simulink model "sampleModel1985"  (R2023a)
settings: Solver=VariableStepAuto  StartTime=0.0  StopTime=10.0  RelTol=1e-3
libraries: hdlsllib x2
settings Model: Creator=user1  LastModifiedBy=user1

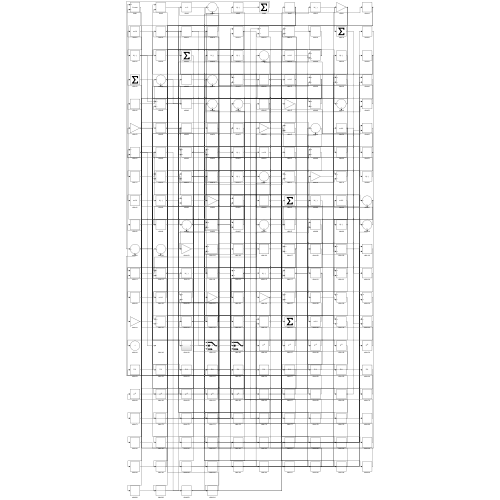
[thumbnail: Simulink's stored preview of the top-level diagram]
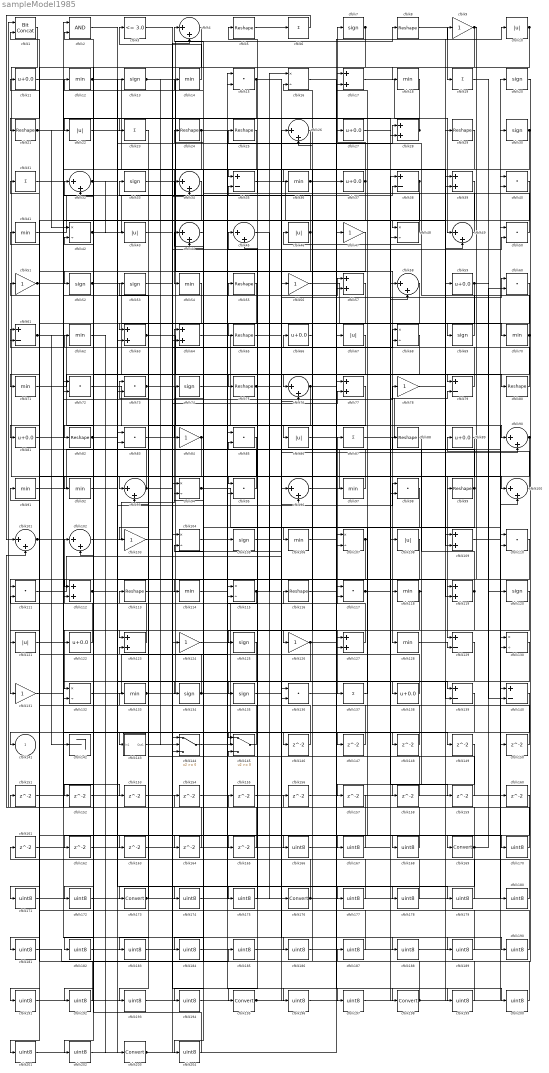
== system sampleModel1985 ==
  cfblk1 : hdlsllib/Logic and Bit Operations/Bit Concat  numInputs=2
  cfblk{10,22,43,46,67,86,108,121} (8 alike) : Abs  SaturateOnIntegerOverflow=off
  cfblk{4,26,32,34,44..45,49,58,76,90,93,96,100..102} (15 alike) : Sum  Inputs=|++
  cfblk{9,47,51,56,78,84,103,124,126,131} (10 alike) : Gain
  cfblk{16,42,48,68,94,104,107,115,130,132} (10 alike) : Product  Inputs=*/  RndMeth=Zero  SaturateOnIntegerOverflow=on
  cfblk{7,13,20,30,33,52..53,69,74,105,120,125,134..135} (14 alike) : Signum
  cfblk{12,14,18,36,41,54,62,70..71,91..92,97,106,114,118,128,133} (17 alike) : MinMax
  cfblk{17,28,39,57,63..64,77,109,112,119,123,127} (12 alike) : Sum
  cfblk{11,27,37,59,66,81,89,122,138} (9 alike) : Bias  Bias=0.0  SaturateOnIntegerOverflow=off
  cfblk{15,40,50,60,72..73,83,85,95,98,110..111,117,136} (14 alike) : DotProduct  OutDataTypeStr=Inherit: Inherit via internal rule
  cfblk{5,8,21,24..25,29,55,65,75,80,82,88,99,113,116} (15 alike) : Reshape
  cfblk{35,38,61,79,129,139..140} (7 alike) : Sum  Inputs=+-
  cfblk{6,19,23,31,87,137} (6 alike) : Sum  Inputs=+
  cfblk142 : Terminator
  cfblk143 : Subsystem
      settings: LibrarySourceBlock=|
      | hdlsllib/Ports &
      | Subsystems/Subsystem
  cfblk144 : Switch  SaturateOnIntegerOverflow=off  InputSameDT=off
  cfblk145 : Switch  SaturateOnIntegerOverflow=off  InputSameDT=off
  cfblk{146..165} (20 alike) : Delay  SampleTime=1
  cfblk{166..168,170..172,174..175,177..194,196..197,199..202,204} (33 alike) : DataTypeConversion  OutDataTypeStr=uint8  SaturateOnIntegerOverflow=off  RndMeth=Floor
  cfblk{169,173,176,195,198,203} (6 alike) : DataTypeConversion  SaturateOnIntegerOverflow=off  RndMeth=Floor
  cfblk2 : Logic  AllPortsSameDT=off  OutDataTypeStr=boolean
  cfblk3 : hdlsllib/Logic and Bit Operations/Compare To Constant  relop=<=  const=3.0  OutDataTypeStr=boolean
  cfblk141 : Outport  VectorParamsAs1DForOutWhenUnconnected=off
  wires:
  cfblk113/1 -> cfblk8/1
  cfblk19/1 -> cfblk120/1
  cfblk83/1 -> cfblk66/1
  cfblk25/1 -> cfblk54/1
  cfblk139/1 -> cfblk141/1
  cfblk5/1 -> cfblk6/1
  cfblk119/1 -> cfblk137/1, cfblk88/1
  cfblk52/1 -> cfblk69/1, cfblk80/1
  cfblk56/1 -> cfblk70/1
  cfblk13/1 -> cfblk128/1, cfblk144/2
  cfblk60/1 -> cfblk79/1
  cfblk61/1 -> cfblk86/1, cfblk143/1(In1), cfblk142/1
  cfblk104/1 -> cfblk198/1
  cfblk99/1 -> cfblk42/2, cfblk147/1
  cfblk122/1 -> cfblk102/1
  cfblk78/1 -> cfblk10/1
  cfblk49/1 -> cfblk12/1
  cfblk1/1 -> cfblk93/1
  cfblk102/1 -> cfblk64/1
  cfblk11/1 -> cfblk35/1
  cfblk117/1 -> cfblk79/2, cfblk149/1
  cfblk46/1 -> cfblk33/1, cfblk75/1, cfblk65/1
  cfblk6/1 -> cfblk101/1
  cfblk118/1 -> cfblk157/1, cfblk158/1
  cfblk77/1 -> cfblk123/1
  cfblk57/1 -> cfblk103/1
  cfblk37/1 -> cfblk7/1, cfblk194/1
  cfblk73/1 -> cfblk178/1, cfblk180/1, cfblk197/1
  cfblk92/1 -> cfblk28/1
  cfblk48/1 -> cfblk4/1
  cfblk127/1 -> cfblk87/1
  cfblk84/1 -> cfblk102/2, cfblk44/2, cfblk191/1
  cfblk120/1 -> cfblk132/1
  cfblk53/1 -> cfblk94/1
  cfblk45/1 -> cfblk176/1
  cfblk137/1 -> cfblk17/1
  cfblk69/1 -> cfblk46/1
  cfblk66/1 -> cfblk106/1
  cfblk63/1 -> cfblk96/1, cfblk35/2
  cfblk111/1 -> cfblk96/2
  cfblk28/1 -> cfblk22/1, cfblk23/1
  cfblk71/1 -> cfblk76/1
  cfblk79/1 -> cfblk44/1
  cfblk76/1 -> cfblk115/2, cfblk9/1
  cfblk144/1 -> cfblk67/1
  cfblk12/1 -> cfblk144/1, cfblk117/2
  cfblk133/1 -> cfblk56/1, cfblk77/2
  cfblk132/1 -> cfblk105/1
  cfblk15/1 -> cfblk82/1, cfblk162/1, cfblk170/1
  cfblk24/1 -> cfblk83/2, cfblk36/1
  cfblk131/1 -> cfblk78/1
  cfblk17/1 -> cfblk49/1
  cfblk88/1 -> cfblk118/1
  cfblk80/1 -> cfblk61/1
  cfblk95/1 -> cfblk32/1
  cfblk134/1 -> cfblk94/2, cfblk73/1, cfblk53/1, cfblk116/1, cfblk32/2
  cfblk70/1 -> cfblk25/1, cfblk95/1
  cfblk31/1 -> cfblk169/1
  cfblk115/1 -> cfblk26/1, cfblk111/2, cfblk16/1
  cfblk96/1 -> cfblk39/1
  cfblk51/1 -> cfblk153/1, cfblk186/1
  cfblk75/1 -> cfblk60/1, cfblk119/2
  cfblk91/1 -> cfblk30/1
  cfblk35/1 -> cfblk49/2
  cfblk124/1 -> cfblk117/1
  cfblk9/1 -> cfblk112/1, cfblk18/1, cfblk119/1
  cfblk103/1 -> cfblk68/1
  cfblk4/1 -> cfblk122/1
  cfblk21/1 -> cfblk48/1, cfblk42/1, cfblk28/2
  cfblk39/1 -> cfblk72/2
  cfblk7/1 -> cfblk64/2, cfblk63/2, cfblk152/1
  cfblk143/1(Out1) -> cfblk68/2
  cfblk72/1 -> cfblk97/1
  cfblk59/1 -> cfblk134/1, cfblk140/2, cfblk63/1
  cfblk90/1 -> cfblk129/1, cfblk111/1
  cfblk33/1 -> cfblk48/2
  cfblk89/1 -> cfblk138/1
  cfblk41/1 -> cfblk4/2
  cfblk58/1 -> cfblk195/1
  cfblk108/1 -> cfblk131/1
  cfblk29/1 -> cfblk84/1
  cfblk26/1 -> cfblk145/1
  cfblk94/1 -> cfblk140/1, cfblk168/1
  cfblk54/1 -> cfblk112/2
  cfblk100/1 -> cfblk89/1
  cfblk101/1 -> cfblk55/1, cfblk34/1
  cfblk82/1 -> cfblk139/1, cfblk172/1
  cfblk85/1 -> cfblk173/1
  cfblk93/1 -> cfblk50/2, cfblk135/1, cfblk41/1
  cfblk34/1 -> cfblk71/1
  cfblk107/1 -> cfblk17/2, cfblk121/1, cfblk174/1
  cfblk121/1 -> cfblk57/1
  cfblk128/1 -> cfblk129/2
  cfblk67/1 -> cfblk92/1
  cfblk22/1 -> cfblk109/1
  cfblk42/1 -> cfblk38/2, cfblk100/1
  cfblk62/1 -> cfblk203/1
  cfblk38/1 -> cfblk125/1, cfblk73/2, cfblk52/1
  cfblk8/1 -> cfblk19/1
  cfblk32/1 -> cfblk43/1, cfblk177/1
  cfblk16/1 -> cfblk107/1
  cfblk3/1 -> cfblk124/1
  cfblk123/1 -> cfblk113/1
  cfblk98/1 -> cfblk114/1
  cfblk145/1 -> cfblk133/1
  cfblk126/1 -> cfblk107/2, cfblk164/1
  cfblk138/1 -> cfblk11/1
  cfblk87/1 -> cfblk59/1
  cfblk129/1 -> cfblk132/2
  cfblk55/1 -> cfblk81/1
  cfblk36/1 -> cfblk109/2, cfblk139/2
  cfblk50/1 -> cfblk5/1
  cfblk14/1 -> cfblk3/1
  cfblk30/1 -> cfblk126/1, cfblk95/2
  cfblk10/1 -> cfblk99/1, cfblk21/1
  cfblk64/1 -> cfblk90/1
  cfblk112/1 -> cfblk98/1, cfblk175/1
  cfblk114/1 -> cfblk127/2
  cfblk97/1 -> cfblk14/1
  cfblk65/1 -> cfblk90/2
  cfblk81/1 -> cfblk146/1
  cfblk146/1 -> cfblk1/2
  cfblk147/1 -> cfblk127/1
  cfblk105/1 -> cfblk148/1
  cfblk148/1 -> cfblk38/1
  cfblk109/1 -> cfblk150/1
  cfblk150/1 -> cfblk26/2
  cfblk151/1 -> cfblk72/1
  cfblk152/1 -> cfblk145/2
  cfblk153/1 -> cfblk76/2
  cfblk154/1 -> cfblk115/1
  cfblk155/1 -> cfblk50/1
  cfblk156/1 -> cfblk98/2
  cfblk157/1 -> cfblk101/2
  cfblk158/1 -> cfblk145/3
  cfblk27/1 -> cfblk159/1
  cfblk159/1 -> cfblk93/2
  cfblk161/1 -> cfblk83/1
  cfblk162/1 -> cfblk34/2
  cfblk68/1 -> cfblk163/1
  cfblk163/1 -> cfblk57/2
  cfblk164/1 -> cfblk61/2
  cfblk140/1 -> cfblk165/1
  cfblk165/1 -> cfblk1/1
  cfblk2/1 -> cfblk166/1
  cfblk166/1 -> cfblk108/1
  cfblk149/1 -> cfblk167/1
  cfblk167/1 -> cfblk2/1
  cfblk168/1 -> cfblk2/2
  cfblk169/1 -> cfblk60/2, cfblk24/1, cfblk183/1
  cfblk170/1 -> cfblk31/1
  cfblk160/1 -> cfblk171/1
  cfblk171/1 -> cfblk15/1
  cfblk172/1 -> cfblk160/1
  cfblk173/1 -> cfblk15/2, cfblk123/2, cfblk27/1
  cfblk174/1 -> cfblk85/1
  cfblk175/1 -> cfblk85/2
  cfblk176/1 -> cfblk156/1, cfblk155/1
  cfblk177/1 -> cfblk45/1
  cfblk178/1 -> cfblk45/2
  cfblk74/1 -> cfblk179/1
  cfblk179/1 -> cfblk51/1
  cfblk180/1 -> cfblk74/1
  cfblk40/1 -> cfblk181/1
  cfblk125/1 -> cfblk182/1
  cfblk182/1 -> cfblk40/1
  cfblk183/1 -> cfblk40/2
  cfblk110/1 -> cfblk184/1
  cfblk184/1 -> cfblk37/1
  cfblk181/1 -> cfblk185/1
  cfblk185/1 -> cfblk110/1
  cfblk186/1 -> cfblk110/2
  cfblk20/1 -> cfblk187/1
  cfblk187/1 -> cfblk161/1
  cfblk106/1 -> cfblk188/1
  cfblk188/1 -> cfblk20/1
  cfblk136/1 -> cfblk189/1
  cfblk189/1 -> cfblk154/1
  cfblk135/1 -> cfblk190/1
  cfblk190/1 -> cfblk136/1
  cfblk191/1 -> cfblk136/2
  cfblk130/1 -> cfblk192/1
  cfblk192/1 -> cfblk151/1
  cfblk23/1 -> cfblk193/1
  cfblk193/1 -> cfblk130/1
  cfblk194/1 -> cfblk130/2
  cfblk195/1 -> cfblk39/2, cfblk29/1
  cfblk43/1 -> cfblk196/1
  cfblk196/1 -> cfblk58/1
  cfblk197/1 -> cfblk58/2
  cfblk198/1 -> cfblk100/2, cfblk16/2, cfblk91/1
  cfblk116/1 -> cfblk199/1
  cfblk199/1 -> cfblk104/1
  cfblk86/1 -> cfblk200/1
  cfblk200/1 -> cfblk104/2
  cfblk47/1 -> cfblk201/1
  cfblk201/1 -> cfblk13/1
  cfblk18/1 -> cfblk202/1
  cfblk202/1 -> cfblk47/1
  cfblk203/1 -> cfblk144/3, cfblk77/1
  cfblk44/1 -> cfblk204/1
  cfblk204/1 -> cfblk62/1

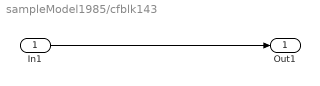
== system sampleModel1985/cfblk143 ==
  In1 : Inport
  Out1 : Outport
  wires:
  In1/1 -> Out1/1
